simulink model "SteadyCamBonito"  (R2015b)
settings: Solver=FixedStepAuto  StartTime=0.0  StopTime=inf  FixedStep=Ts  RelTol=1e-3
InitFcn:
  | InitSteady;
values from neighbouring files (symbols this model uses):
  Deg2Rad = pi/180    (= 0.0174532925199)    [InitSteady.m]
  GainGyro = 90/12000    (= 0.0075)    [InitSteady.m]
  HighValFilter = 0.99    [InitSteady.m]
  InitTime = 2.9    [InitSteady.m]
  LowValFilter = 0.01    [InitSteady.m]
  PID_Activator = 35    [InitSteady.m]
  Rad2Deg = 180/pi    (= 57.2957795131)    [InitSteady.m]
  Ts = 0.03    [InitSteady.m]
undefined symbols (not defined in the file or in its folder): DiscIntNeverNeededParam
libraries: simulink x4, RASPlib x2
settings Model: SimulationMode=external  ExtModeTrigDuration=2  Creator=Simón  LastModifiedBy=Simón
settings OptimizationCC: OptimizeModelRefInitCode=on  LifeSpan=Inf  MaxStackSize=64
settings HardwareCC: ProdBitPerInt=16  ProdBitPerPointer=16  ProdLargestAtomicFloat=None  ProdWordSize=8  ProdHWDeviceType=Atmel->AVR
settings RTWCC: SystemTargetFile=ert.tlc  TemplateMakefile=ert_default_tmf  Description=Embedded Coder  Toolchain=Arduino AVR v1.6.1  BuildConfiguration=Faster Runs
settings CodeAppCC: IgnoreCustomStorageClasses=off
settings ERTTargetCC: SupportContinuousTime=on  SupportVariableSizeSignals=on

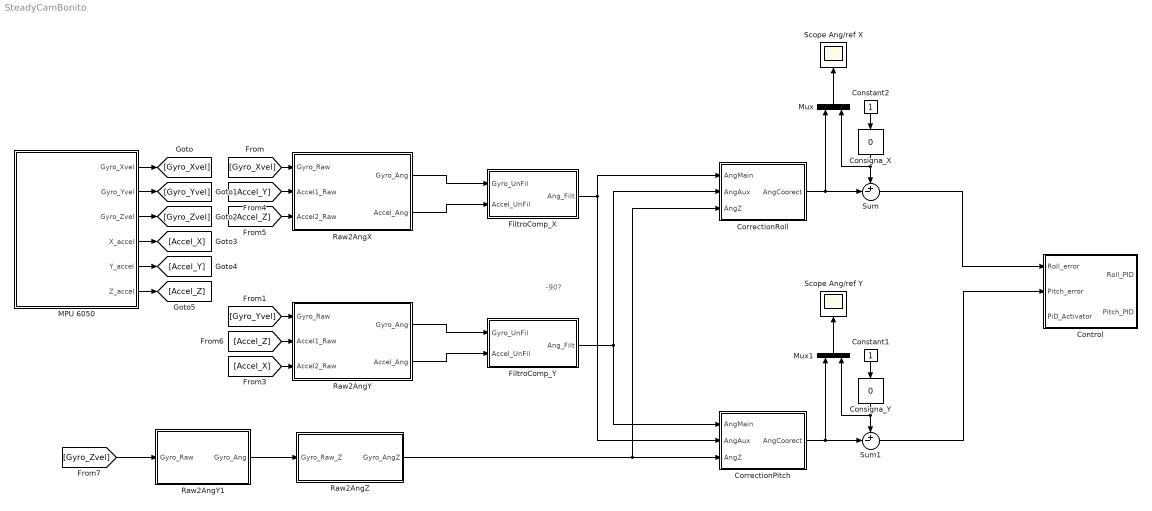
== system SteadyCamBonito ==
  note: -90?
  Consigna_X : simulink/Math Operations/Slider Gain  low=-25  gain=0  high=35
  Consigna_Y : simulink/Math Operations/Slider Gain  low=-25  gain=0  high=35
  Constant1 : Constant
  Constant2 : Constant
  Control : Subsystem
  CorrectionPitch : Subsystem
  CorrectionRoll : Subsystem
  FiltroComp_X : Subsystem
  FiltroComp_Y : Subsystem
  MPU 6050 : Subsystem
  Mux : Mux  Inputs=2
  Mux1 : Mux  Inputs=2
  Raw2AngX : Subsystem
  Raw2AngY : Subsystem
  Raw2AngY1 : Subsystem
  Raw2AngZ : Subsystem
  Scope Ang/ref X : Scope
  Scope Ang/ref Y : Scope
  Sum : Sum  Inputs=+-|
  Sum1 : Sum  Inputs=+-|
  wires:
  CorrectionRoll/1(AngCoorect) -> Mux/1, Sum/2
  Constant2/1 -> Consigna_X/1
  Consigna_X/1 -> Mux/2, Sum/1
  Raw2AngX/1(Gyro_Ang) -> FiltroComp_X/1(Gyro_UnFil)
  Raw2AngX/2(Accel_Ang) -> FiltroComp_X/2(Accel_UnFil)
  Mux/1 -> Scope Ang/ref X/1
  Raw2AngY/1(Gyro_Ang) -> FiltroComp_Y/1(Gyro_UnFil)
  Raw2AngY/2(Accel_Ang) -> FiltroComp_Y/2(Accel_UnFil)
  CorrectionPitch/1(AngCoorect) -> Sum1/2, Mux1/1
  Constant1/1 -> Consigna_Y/1
  Consigna_Y/1 -> Sum1/1, Mux1/2
  Mux1/1 -> Scope Ang/ref Y/1
  FiltroComp_X/1(Ang_Filt) -> CorrectionPitch/2(AngAux), CorrectionRoll/1(AngMain)
  FiltroComp_Y/1(Ang_Filt) -> CorrectionRoll/2(AngAux), CorrectionPitch/1(AngMain)
  Raw2AngZ/1("Gyro_AngZ ") -> CorrectionRoll/3(AngZ), CorrectionPitch/3(AngZ)
  Sum/1 -> Control/1(Roll_error)
  Sum1/1 -> Control/2(Pitch_error)
  MPU 6050/1("Gyro_Xvel ") -> [Gyro_Xvel]
  [Gyro_Xvel] -> Raw2AngX/1(Gyro_Raw)
  MPU 6050/2(Gyro_Yvel) -> [Gyro_Yvel]
  MPU 6050/3(Gyro_Zvel) -> [Gyro_Zvel]
  [Gyro_Yvel] -> Raw2AngY/1(Gyro_Raw)
  Raw2AngY1/1(Gyro_Ang) -> Raw2AngZ/1(Gyro_Raw_Z)
  MPU 6050/4(X_accel) -> [Accel_X]
  [Accel_X] -> Raw2AngY/3(Accel2_Raw)
  MPU 6050/5(Y_accel) -> [Accel_Y]
  [Accel_Y] -> Raw2AngX/2(Accel1_Raw)
  MPU 6050/6(Z_accel) -> [Accel_Z]
  [Accel_Z] -> Raw2AngX/3(Accel2_Raw)
  [Accel_Z] -> Raw2AngY/2(Accel1_Raw)
  [Gyro_Zvel] -> Raw2AngY1/1(Gyro_Raw)

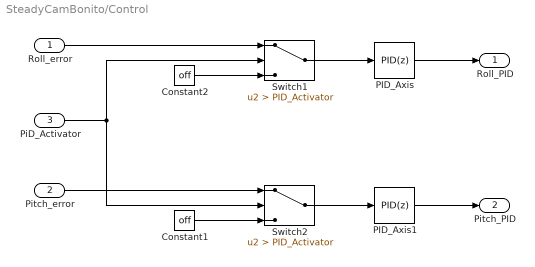
== system SteadyCamBonito/Control ==
  Roll_error : Inport
  Pitch_error : Inport  Port=2
  PiD_Activator : Inport  Port=3
  Constant1 : Constant  Value=off
  Constant2 : Constant  Value=off
  PID_Axis : simulink/Continuous/PID Controller  Controller=PID  TimeDomain=Discrete-time  SampleTime=-1  IntegratorMethod=Forward Euler  FilterMethod=Forward Euler  Form=Parallel  UseFilter=off  ControllerParametersSource=internal  P=0.51  I=0.425  D=0.106  N=30  InitialConditionSource=internal  InitialConditionForIntegrator=0  InitialConditionForFilter=0  ExternalReset=none  LimitOutput=off  UpperSaturationLimit=inf  LowerSaturationLimit=-inf  LinearizeAsGain=off  AntiWindupMode=none  Kb=1  TrackingMode=off  Kt=1  PParamMin=[]  PParamMax=[]  IParamMin=[]  IParamMax=[]  DParamMin=[]  DParamMax=[]  NParamMin=[]  NParamMax=[]  KbParamMin=[]  KbParamMax=[]  KtParamMin=[]  KtParamMax=[]  POutMin=[]  POutMax=[]  IOutMin=[]  IOutMax=[]  DOutMin=[]  DOutMax=[]  NOutMin=[]  NOutMax=[]  KbOutMin=[]  KbOutMax=[]  KtOutMin=[]  KtOutMax=[]  IntegratorOutMin=[]  IntegratorOutMax=[]  FilterOutMin=[]  FilterOutMax=[]  SumOutMin=[]  SumOutMax=[]  SumI1OutMin=[]  SumI1OutMax=[]  SumI2OutMin=[]  SumI2OutMax=[]  SumI3OutMin=[]  SumI3OutMax=[]  SumDOutMin=[]  SumDOutMax=[]  SaturationOutMin=[]  SaturationOutMax=[]  IntegratorContinuousStateAttributes=''  IntegratorStateMustResolveToSignalObject=off  IntegratorRTWStateStorageClass=Auto  FilterContinuousStateAttributes=''  FilterStateMustResolveToSignalObject=off  FilterRTWStateStorageClass=Auto  DifferentiatorICPrevScaledInput=0  DifferentiatorOutMin=[]  DifferentiatorOutMax=[]
  PID_Axis1 : simulink/Continuous/PID Controller  Controller=PID  TimeDomain=Discrete-time  SampleTime=-1  IntegratorMethod=Forward Euler  FilterMethod=Forward Euler  Form=Parallel  UseFilter=off  ControllerParametersSource=internal  P=0.51  I=0.425  D=0.106  N=30  InitialConditionSource=internal  InitialConditionForIntegrator=0  InitialConditionForFilter=0  ExternalReset=none  LimitOutput=off  UpperSaturationLimit=inf  LowerSaturationLimit=-inf  LinearizeAsGain=off  AntiWindupMode=none  Kb=1  TrackingMode=off  Kt=1  PParamMin=[]  PParamMax=[]  IParamMin=[]  IParamMax=[]  DParamMin=[]  DParamMax=[]  NParamMin=[]  NParamMax=[]  KbParamMin=[]  KbParamMax=[]  KtParamMin=[]  KtParamMax=[]  POutMin=[]  POutMax=[]  IOutMin=[]  IOutMax=[]  DOutMin=[]  DOutMax=[]  NOutMin=[]  NOutMax=[]  KbOutMin=[]  KbOutMax=[]  KtOutMin=[]  KtOutMax=[]  IntegratorOutMin=[]  IntegratorOutMax=[]  FilterOutMin=[]  FilterOutMax=[]  SumOutMin=[]  SumOutMax=[]  SumI1OutMin=[]  SumI1OutMax=[]  SumI2OutMin=[]  SumI2OutMax=[]  SumI3OutMin=[]  SumI3OutMax=[]  SumDOutMin=[]  SumDOutMax=[]  SaturationOutMin=[]  SaturationOutMax=[]  IntegratorContinuousStateAttributes=''  IntegratorStateMustResolveToSignalObject=off  IntegratorRTWStateStorageClass=Auto  FilterContinuousStateAttributes=''  FilterStateMustResolveToSignalObject=off  FilterRTWStateStorageClass=Auto  DifferentiatorICPrevScaledInput=0  DifferentiatorOutMin=[]  DifferentiatorOutMax=[]
  Switch1 : Switch  Criteria=u2 > Threshold  Threshold=PID_Activator
  Switch2 : Switch  Criteria=u2 > Threshold  Threshold=PID_Activator
  Roll_PID : Outport
  Pitch_PID : Outport  Port=2
  wires:
  PID_Axis/1 -> Roll_PID/1
  Switch1/1 -> PID_Axis/1
  PiD_Activator/1 -> Switch1/2, Switch2/2
  Constant2/1 -> Switch1/3
  Roll_error/1 -> Switch1/1
  Switch2/1 -> PID_Axis1/1
  Constant1/1 -> Switch2/3
  Pitch_error/1 -> Switch2/1
  PID_Axis1/1 -> Pitch_PID/1

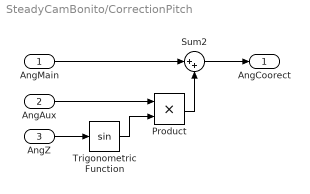
== system SteadyCamBonito/CorrectionPitch ==
  AngMain : Inport
  AngAux : Inport  Port=2
  AngZ : Inport  Port=3
  Product : Product
  Sum2 : Sum  Inputs=|++
  Trigonometric Function : Trigonometry
  AngCoorect : Outport
  wires:
  Trigonometric Function/1 -> Product/2
  Product/1 -> Sum2/2
  AngMain/1 -> Sum2/1
  AngZ/1 -> Trigonometric Function/1
  Sum2/1 -> AngCoorect/1
  AngAux/1 -> Product/1

== system SteadyCamBonito/CorrectionRoll ==
  AngMain : Inport
  AngAux : Inport  Port=2
  AngZ : Inport  Port=3
  Product : Product
  Sum2 : Sum  Inputs=|++
  Trigonometric Function : Trigonometry
  AngCoorect : Outport
  wires:
  AngAux/1 -> Product/1
  Sum2/1 -> AngCoorect/1
  AngZ/1 -> Trigonometric Function/1
  AngMain/1 -> Sum2/1
  Product/1 -> Sum2/2
  Trigonometric Function/1 -> Product/2

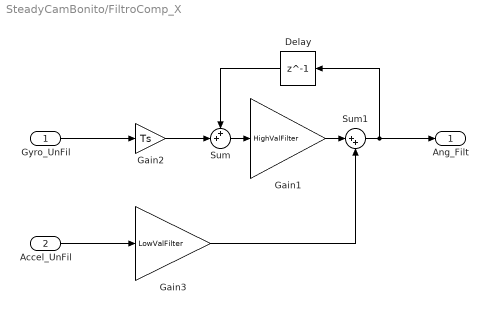
== system SteadyCamBonito/FiltroComp_X ==
  Gyro_UnFil : Inport
  Accel_UnFil : Inport  Port=2
  Delay : Delay  DelayLength=1  InitialCondition=0
  Gain1 : Gain  Gain=HighValFilter
  Gain2 : Gain  Gain=Ts
  Gain3 : Gain  Gain=LowValFilter
  Sum : Sum  Inputs=++|
  Sum1 : Sum  Inputs=|++
  Ang_Filt : Outport
  wires:
  Gain3/1 -> Sum1/2
  Gyro_UnFil/1 -> Gain2/1
  Sum1/1 -> Ang_Filt/1, Delay/1
  Gain1/1 -> Sum1/1
  Accel_UnFil/1 -> Gain3/1
  Sum/1 -> Gain1/1
  Delay/1 -> Sum/1
  Gain2/1 -> Sum/2

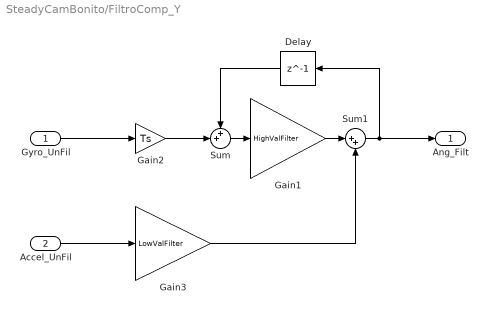
== system SteadyCamBonito/FiltroComp_Y ==
  Gyro_UnFil : Inport
  Accel_UnFil : Inport  Port=2
  Delay : Delay  DelayLength=1  InitialCondition=0
  Gain1 : Gain  Gain=HighValFilter
  Gain2 : Gain  Gain=Ts
  Gain3 : Gain  Gain=LowValFilter
  Sum : Sum  Inputs=++|
  Sum1 : Sum  Inputs=|++
  Ang_Filt : Outport
  wires:
  Gain2/1 -> Sum/2
  Delay/1 -> Sum/1
  Sum/1 -> Gain1/1
  Accel_UnFil/1 -> Gain3/1
  Gain1/1 -> Sum1/1
  Sum1/1 -> Delay/1, Ang_Filt/1
  Gyro_UnFil/1 -> Gain2/1
  Gain3/1 -> Sum1/2

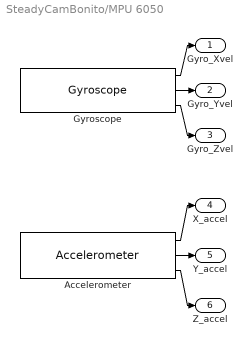
== system SteadyCamBonito/MPU 6050 ==
  Accelerometer : RASPlib/Accelerometer  SimulateUsing=Code generation
  Gyroscope : RASPlib/Gyroscope  DLPFmode=0
  "Gyro_Xvel " : Outport
  Gyro_Yvel : Outport  Port=2
  Gyro_Zvel : Outport  Port=3
  X_accel : Outport  Port=4
  Y_accel : Outport  Port=5
  Z_accel : Outport  Port=6
  wires:
  Accelerometer/2 -> Y_accel/1
  Accelerometer/3 -> Z_accel/1
  Gyroscope/1 -> "Gyro_Xvel "/1
  Gyroscope/2 -> Gyro_Yvel/1
  Gyroscope/3 -> Gyro_Zvel/1
  Accelerometer/1 -> X_accel/1

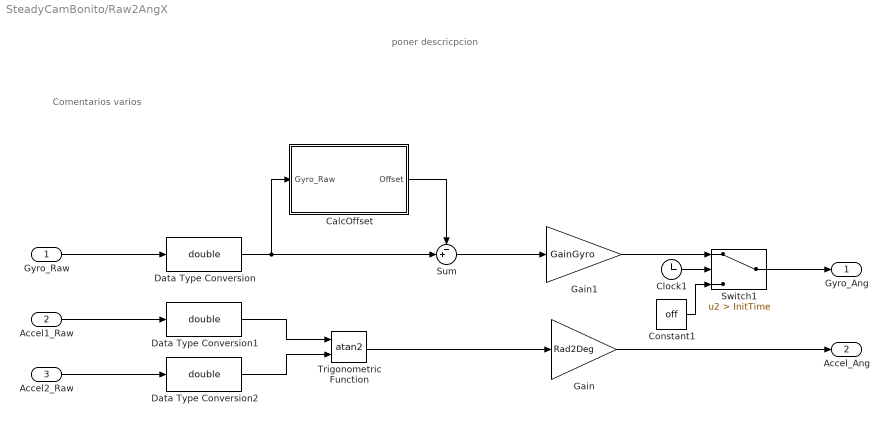
== system SteadyCamBonito/Raw2AngX ==
  note: poner descricpcion
  note: Comentarios varios
  Gyro_Raw : Inport
  Accel1_Raw : Inport  Port=2
  Accel2_Raw : Inport  Port=3
  CalcOffset : Subsystem
  Clock1 : Clock
  Constant1 : Constant  Value=off
  Data Type Conversion : DataTypeConversion  OutDataTypeStr=double
  Data Type Conversion1 : DataTypeConversion  OutDataTypeStr=double
  Data Type Conversion2 : DataTypeConversion  OutDataTypeStr=double
  Gain : Gain  Gain=Rad2Deg
  Gain1 : Gain  Gain=GainGyro
  Sum : Sum  Inputs=-+|
  Switch1 : Switch  Criteria=u2 > Threshold  Threshold=InitTime
  Trigonometric Function : Trigonometry  Operator=atan2
  Gyro_Ang : Outport
  Accel_Ang : Outport  Port=2
  wires:
  Accel2_Raw/1 -> Data Type Conversion2/1
  Constant1/1 -> Switch1/3
  Gain1/1 -> Switch1/1
  Gyro_Raw/1 -> Data Type Conversion/1
  Trigonometric Function/1 -> Gain/1
  Switch1/1 -> Gyro_Ang/1
  Clock1/1 -> Switch1/2
  Data Type Conversion1/1 -> Trigonometric Function/1
  Data Type Conversion2/1 -> Trigonometric Function/2
  Accel1_Raw/1 -> Data Type Conversion1/1
  Gain/1 -> Accel_Ang/1
  Sum/1 -> Gain1/1
  Data Type Conversion/1 -> CalcOffset/1(Gyro_Raw), Sum/2
  CalcOffset/1(Offset) -> Sum/1

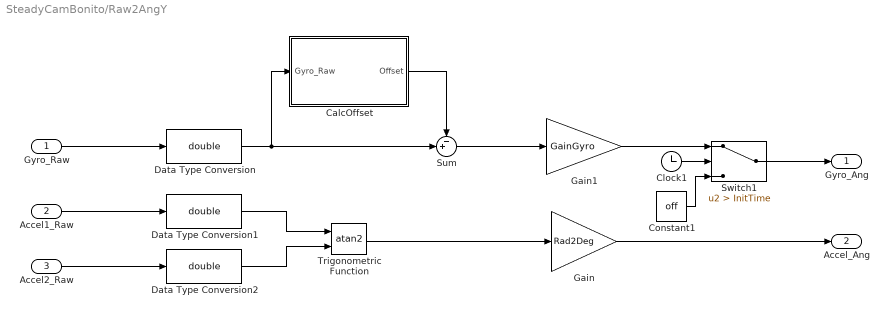
== system SteadyCamBonito/Raw2AngY ==
  Gyro_Raw : Inport
  Accel1_Raw : Inport  Port=2
  Accel2_Raw : Inport  Port=3
  CalcOffset : Subsystem
  Clock1 : Clock
  Constant1 : Constant  Value=off
  Data Type Conversion : DataTypeConversion  OutDataTypeStr=double
  Data Type Conversion1 : DataTypeConversion  OutDataTypeStr=double
  Data Type Conversion2 : DataTypeConversion  OutDataTypeStr=double
  Gain : Gain  Gain=Rad2Deg
  Gain1 : Gain  Gain=GainGyro
  Sum : Sum  Inputs=-+|
  Switch1 : Switch  Criteria=u2 > Threshold  Threshold=InitTime
  Trigonometric Function : Trigonometry  Operator=atan2
  Gyro_Ang : Outport
  Accel_Ang : Outport  Port=2
  wires:
  CalcOffset/1(Offset) -> Sum/1
  Data Type Conversion/1 -> Sum/2, CalcOffset/1(Gyro_Raw)
  Sum/1 -> Gain1/1
  Gain/1 -> Accel_Ang/1
  Accel1_Raw/1 -> Data Type Conversion1/1
  Data Type Conversion2/1 -> Trigonometric Function/2
  Data Type Conversion1/1 -> Trigonometric Function/1
  Clock1/1 -> Switch1/2
  Switch1/1 -> Gyro_Ang/1
  Trigonometric Function/1 -> Gain/1
  Gyro_Raw/1 -> Data Type Conversion/1
  Gain1/1 -> Switch1/1
  Constant1/1 -> Switch1/3
  Accel2_Raw/1 -> Data Type Conversion2/1

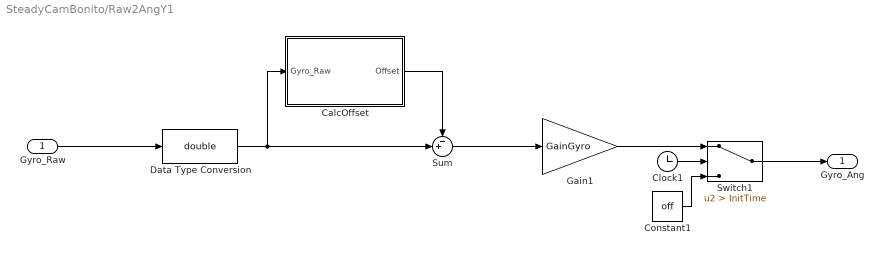
== system SteadyCamBonito/Raw2AngY1 ==
  Gyro_Raw : Inport
  CalcOffset : Subsystem
  Clock1 : Clock
  Constant1 : Constant  Value=off
  Data Type Conversion : DataTypeConversion  OutDataTypeStr=double
  Gain1 : Gain  Gain=GainGyro
  Sum : Sum  Inputs=-+|
  Switch1 : Switch  Criteria=u2 > Threshold  Threshold=InitTime
  Gyro_Ang : Outport
  wires:
  Constant1/1 -> Switch1/3
  Gain1/1 -> Switch1/1
  Gyro_Raw/1 -> Data Type Conversion/1
  Switch1/1 -> Gyro_Ang/1
  Clock1/1 -> Switch1/2
  Sum/1 -> Gain1/1
  Data Type Conversion/1 -> CalcOffset/1(Gyro_Raw), Sum/2
  CalcOffset/1(Offset) -> Sum/1

== system SteadyCamBonito/Raw2AngZ ==
  Gyro_Raw_Z : Inport
  Data Type Conversion3 : DataTypeConversion  OutDataTypeStr=double
  Discrete-Time Integrator : DiscreteIntegrator  InitialConditionSetting=State (most efficient)  SampleTime=Ts  ICPrevOutput=DiscIntNeverNeededParam  ICPrevScaledInput=DiscIntNeverNeededParam
  Gain : Gain  Gain=Deg2Rad
  "Gyro_AngZ " : Outport
  wires:
  Discrete-Time Integrator/1 -> Data Type Conversion3/1
  Gain/1 -> "Gyro_AngZ "/1
  Gyro_Raw_Z/1 -> Discrete-Time Integrator/1
  Data Type Conversion3/1 -> Gain/1

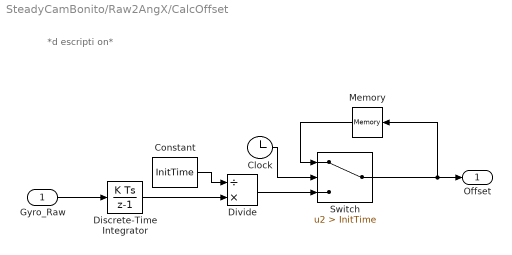
== system SteadyCamBonito/Raw2AngX/CalcOffset ==
  note: *d escripti on*
  Gyro_Raw : Inport
  Clock : Clock
  Constant : Constant  Value=InitTime
  Discrete-Time Integrator : DiscreteIntegrator  InitialConditionSetting=State (most efficient)  SampleTime=Ts  ICPrevOutput=DiscIntNeverNeededParam  ICPrevScaledInput=DiscIntNeverNeededParam
  Divide : Product  Inputs=/*
  Memory : Memory
  Switch : Switch  Criteria=u2 > Threshold  Threshold=InitTime
  Offset : Outport
  wires:
  Divide/1 -> Switch/3
  Discrete-Time Integrator/1 -> Divide/2
  Memory/1 -> Switch/1
  Constant/1 -> Divide/1
  Switch/1 -> Memory/1, Offset/1
  Clock/1 -> Switch/2
  Gyro_Raw/1 -> Discrete-Time Integrator/1

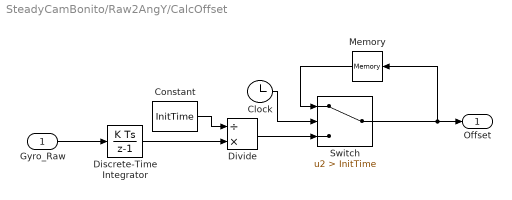
== system SteadyCamBonito/Raw2AngY/CalcOffset ==
  Gyro_Raw : Inport
  Clock : Clock
  Constant : Constant  Value=InitTime
  Discrete-Time Integrator : DiscreteIntegrator  InitialConditionSetting=State (most efficient)  SampleTime=Ts  ICPrevOutput=DiscIntNeverNeededParam  ICPrevScaledInput=DiscIntNeverNeededParam
  Divide : Product  Inputs=/*
  Memory : Memory
  Switch : Switch  Criteria=u2 > Threshold  Threshold=InitTime
  Offset : Outport
  wires:
  Gyro_Raw/1 -> Discrete-Time Integrator/1
  Clock/1 -> Switch/2
  Switch/1 -> Offset/1, Memory/1
  Constant/1 -> Divide/1
  Memory/1 -> Switch/1
  Discrete-Time Integrator/1 -> Divide/2
  Divide/1 -> Switch/3

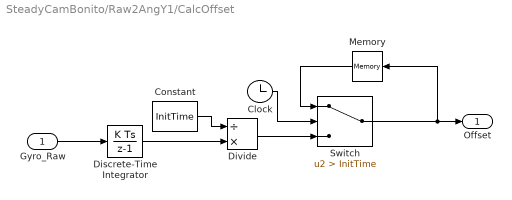
== system SteadyCamBonito/Raw2AngY1/CalcOffset ==
  Gyro_Raw : Inport
  Clock : Clock
  Constant : Constant  Value=InitTime
  Discrete-Time Integrator : DiscreteIntegrator  InitialConditionSetting=State (most efficient)  SampleTime=Ts  ICPrevOutput=DiscIntNeverNeededParam  ICPrevScaledInput=DiscIntNeverNeededParam
  Divide : Product  Inputs=/*
  Memory : Memory
  Switch : Switch  Criteria=u2 > Threshold  Threshold=InitTime
  Offset : Outport
  wires:
  Divide/1 -> Switch/3
  Discrete-Time Integrator/1 -> Divide/2
  Memory/1 -> Switch/1
  Constant/1 -> Divide/1
  Switch/1 -> Memory/1, Offset/1
  Clock/1 -> Switch/2
  Gyro_Raw/1 -> Discrete-Time Integrator/1
